simulink model "IEEE_14bus"  (R2021a)
settings: Solver=VariableStepAuto  StartTime=0.0  StopTime=16  RelTol=1e-3
undefined symbols (not defined in the file): c, cost, Discrete, linsys1, M, Mdot, Req, THeater, Time, TinIC
libraries: spsThreePhaseVIMeasurementLib x52, spsThreePhasePISectionLineLib x20, spsPMUPLLBasedPositiveSequenceLib x14, spsThreePhaseSeriesRLCLoadLib x12, spsThreePhaseTransformerTwoWindingsLib x6, simulink x6, spsThreePhaseBreakerLib x4, rllib x3, simulink_extras x3, eeStairGenerator x3, spsThreePhaseSourceLib x3, spsSynchronousMachinepuStandardLib x3
(part 2 of 3)

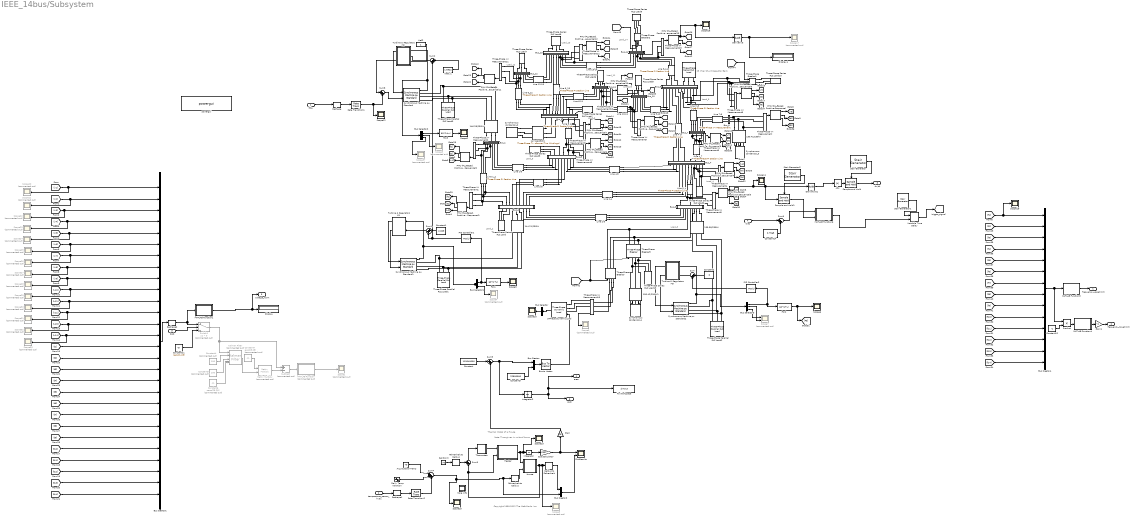
== system IEEE_14bus/Subsystem ==
  note: 25 MVar Shunt
      | Capacitor Bank
  note: Load_9
  note: Copyright 1990-2012 The MathWorks, Inc.
  note: Load_10
  note: Load_14
  note: Load_13
  note: Load_5
  note: Load_4
  note: Thermal Model of a House
  note: Load_2
  note: Load_3
  note: Load_12
  note: Load_11
  note: Note: Time given in units of hours
  note: Load_6
  fdia : Inport
  temperature_sensor_hvac : Inport  Port=2
  DoS : Inport  Port=3
  bias : Inport  Port=4
  " " : spsThreePhaseSeriesRLCLoadLib/Three-Phase Series RLC Load  LConnTagsString=A|B|C  Configuration=Y (grounded)  NominalVoltage=230e3  Vabc=[1e3 1e3 1e3]  Vabcp=[1e3 1e3 1e3]  NominalFrequency=60  UnbalancedPower=off  ActivePower=0  InductivePower=0  CapacitivePower=25e6  Pabc=[10e3 9e3 11e3]  QLabc=[100 90 110]  QCabc=[100 90 110]  Pabcp=[10e3 9e3 11e3]  QLabcp=[100 90 110]  QCabcp=[100 90 110]  Measurements=None  LoadType=constant Z
  139.38/230kV : spsThreePhaseTransformerTwoWindingsLib/Three-Phase Transformer (Two Windings)  Winding1Connection=Yg  Winding2Connection=Yg  CoreType=Three single-phase transformers  SetSaturation=off  Hysteresis=off  DataFile='hysteresis'  SetInitialFlux=off  Measurements=None  UNITS=pu  NominalPower=[ 120e6 , 60 ]  Winding1=[139.38e3 , 0.002 , 0.08 ]  Winding2=[ 230e3 , 0.002 , 0.08 ]  Rm=500  Lm=500  L0=0.5  Saturation=[ 0,0 ; 0.0024,1.2 ; 1.0,1.52 ]  InitialFluxes=[ 0.8 , -0.8 , 0.7 ]  BreakLoop=off  DiscreteSolver=Trapezoidal iterative  DataType=off  TransfoNumber=1
  144.21/230kV : spsThreePhaseTransformerTwoWindingsLib/Three-Phase Transformer (Two Windings)  Winding1Connection=Yg  Winding2Connection=Yg  CoreType=Three single-phase transformers  SetSaturation=off  Hysteresis=off  DataFile='hysteresis'  SetInitialFlux=off  Measurements=None  UNITS=pu  NominalPower=[ 120e6 , 60 ]  Winding1=[144.21e3 , 0.002 , 0.08 ]  Winding2=[ 230e3 , 0.002 , 0.08 ]  Rm=500  Lm=500  L0=0.5  Saturation=[ 0,0 ; 0.0024,1.2 ; 1.0,1.52 ]  InitialFluxes=[ 0.8 , -0.8 , 0.7 ]  BreakLoop=off  DiscreteSolver=Trapezoidal iterative  DataType=off  TransfoNumber=1
  146.28/230kV : spsThreePhaseTransformerTwoWindingsLib/Three-Phase Transformer (Two Windings)  Winding1Connection=Yg  Winding2Connection=Yg  CoreType=Three single-phase transformers  SetSaturation=off  Hysteresis=off  DataFile='hysteresis'  SetInitialFlux=off  Measurements=None  UNITS=pu  NominalPower=[ 120e6 , 60 ]  Winding1=[146.28e3 , 0.002 , 0.08 ]  Winding2=[ 230e3 , 0.002 , 0.08 ]  Rm=500  Lm=500  L0=0.5  Saturation=[ 0,0 ; 0.0024,1.2 ; 1.0,1.52 ]  InitialFluxes=[ 0.8 , -0.8 , 0.7 ]  BreakLoop=off  DiscreteSolver=Trapezoidal iterative  DataType=off  TransfoNumber=1
  147.66/230kV : spsThreePhaseTransformerTwoWindingsLib/Three-Phase Transformer (Two Windings)  Winding1Connection=Yg  Winding2Connection=Yg  CoreType=Three single-phase transformers  SetSaturation=off  Hysteresis=off  DataFile='hysteresis'  SetInitialFlux=off  Measurements=None  UNITS=pu  NominalPower=[ 120e6 , 60 ]  Winding1=[147.66e3 , 0.002 , 0.08 ]  Winding2=[ 230e3 , 0.002 , 0.08 ]  Rm=500  Lm=500  L0=0.5  Saturation=[ 0,0 ; 0.0024,1.2 ; 1.0,1.52 ]  InitialFluxes=[ 0.8 , -0.8 , 0.7 ]  BreakLoop=off  DiscreteSolver=Trapezoidal iterative  DataType=off  TransfoNumber=1
  150.42/230kV : spsThreePhaseTransformerTwoWindingsLib/Three-Phase Transformer (Two Windings)  Winding1Connection=Yg  Winding2Connection=Yg  CoreType=Three single-phase transformers  SetSaturation=off  Hysteresis=off  DataFile='hysteresis'  SetInitialFlux=off  Measurements=None  UNITS=pu  NominalPower=[ 120e6 , 60 ]  Winding1=[150.42e3 , 0.002 , 0.08 ]  Winding2=[ 230e3 , 0.002 , 0.08 ]  Rm=500  Lm=500  L0=0.5  Saturation=[ 0,0 ; 0.0024,1.2 ; 1.0,1.52 ]  InitialFluxes=[ 0.8 , -0.8 , 0.7 ]  BreakLoop=off  DiscreteSolver=Trapezoidal iterative  DataType=off  TransfoNumber=1
  150.42/230kV1 : spsThreePhaseTransformerTwoWindingsLib/Three-Phase Transformer (Two Windings)  Winding1Connection=Yg  Winding2Connection=Yg  CoreType=Three single-phase transformers  SetSaturation=off  Hysteresis=off  DataFile='hysteresis'  SetInitialFlux=off  Measurements=None  UNITS=pu  NominalPower=[ 120e6 , 60 ]  Winding1=[150.42e3 , 0.002 , 0.08 ]  Winding2=[ 230e3 , 0.002 , 0.08 ]  Rm=500  Lm=500  L0=0.5  Saturation=[ 0,0 ; 0.0024,1.2 ; 1.0,1.52 ]  InitialFluxes=[ 0.8 , -0.8 , 0.7 ]  BreakLoop=off  DiscreteSolver=Trapezoidal iterative  DataType=off  TransfoNumber=1
  3-Phase Dynamic Load : spsThreePhaseDynamicLoadLib/Three-Phase Dynamic Load  NominalVoltage=[ (217684)*1 60 ]  ActiveReactivePowers=[113.04e6 22.8e6]  PositiveSequence=[0.98441 -1.41063]  ExternalControl=on  NpNq="[1  1]"  TimeConstants="[0  0  0  0]"  MinimumVoltage=0.7  Tfilter=1e-4  LoadFlowParameters=[4 50000000 0 0 25000000]
      settings: SourceProductBaseCode=PS
  Abs : Abs
  Avg Outdoor Temp : Constant  Value=70
  Bus Creator : BusCreator  Inputs=2
  Bus Creator1 : BusCreator  Inputs=28
  Bus Creator2 : BusCreator  Inputs=2
  Bus Creator4 : BusCreator  Inputs=14
  Bus Selector : BusSelector  OutputSignals=Positive-sequence voltage V (pu)
  Bus Selector1 : BusSelector  OutputSignals="Mechanical.Rotor speed deviation  dw (pu),Mechanical.Electrical power  Pe (pu)"
  Bus Selector2 : BusSelector  OutputSignals="Mechanical.Rotor speed deviation  dw (pu),Mechanical.Electrical power  Pe (pu),dq0 components.Stator current  id (pu)"
  Bus Selector3 : BusSelector  OutputSignals="Mechanical.Rotor speed deviation  dw (pu),Mechanical.Electrical power  Pe (pu),Output active power   Peo (pu)"
  Bus to Vector : BusToVector
  Bus_1 : Subsystem
  Bus_10 : Subsystem
  Bus_11 : Subsystem
  Bus_12 : Subsystem
  Bus_13 : Subsystem
  Bus_14 : Subsystem
  Bus_2 : Subsystem
  Bus_3 : Subsystem
  Bus_4 : Subsystem
  Bus_5 : Subsystem
  Bus_6 : Subsystem
  Bus_7 : Subsystem
  Bus_8 : spsThreePhaseVIMeasurementLib/Three-Phase V-I Measurement  VoltageMeasurement=phase-to-phase  SetLabelV=on  LabelV=VB_8  Vpu=off  VpuLL=off  CurrentMeasurement=yes  SetLabelI=on  LabelI=IB_8  Ipu=off  Pbase=100e6  Vbase=500e3  OutputType=Complex  PhasorSimulation=off  PSBequivalent=0
  Bus_9 : Subsystem
  Celsius to Fahrenheit : simulink_extras/Transformations/Celsius to Fahrenheit
      settings: SourceProductBaseCode=SL
  Constant : Constant  Value=113040000
  Constant1 : Constant  Value=2.009
  Constant11 : Constant  Value=zeros(1,28)
  Constant12 : Constant  Value=-1
  Constant14 : Constant  Value=0.75e5
  Constant2 : Constant  Value=0
  Constant3 : Constant  Value=22800000
  Constant4 : Constant  Commented=on  Value=100
  Constant5 : Constant  Commented=on  Value=100
  Constant6 : Constant  Commented=on  Value=zeros(28,28)
  Constant7 : Constant  Commented=on  Value=eye(28,28)
  Cost Calculator : Gain  Gain=cost  SaturateOnIntegerOverflow=on  OutDataTypeStr=Inherit: Same as input  ParamDataTypeStr=Inherit: Same as input
  Daily Temp Variation : Sin  Amplitude=-7  Frequency=2*pi/120  SampleTime=0
  Derivative : Derivative
  Derivative1 : Derivative
  Display : Display
  Display4 : Display
  Fahrenheit to Celsius : simulink_extras/Transformations/Fahrenheit to Celsius
      settings: SourceProductBaseCode=SL
  "Fahrenheit to Celsius " : simulink_extras/Transformations/Fahrenheit to Celsius
      settings: SourceProductBaseCode=SL
  Fcn1 : Fcn  Expr=60*(1+u)
  Fcn2 : Fcn  Expr=60*(1+u)
  Fcn3 : Fcn  Expr=60*(1+u)
  Gain : Gain  Gain=9e7
  Gain1 : Gain  Gain=-1
  Heater : Subsystem
  House : Subsystem
      mask Display: image(fullfile(matlabroot,'toolbox','simulink','simdemos','simgeneral','images','HouseHeatHousePix.svg'))
  Integrator : Integrator  InitialCondition=TinIC
  Integrator2 : Integrator
  Kalman Filter : ctrlSharedLib/Kalman Filter  Commented=on  TimeDomain=Discrete-Time  UseCurrentEstimator=on  ModelSource=Individual A, B, C, D matrices  ModelSourceVariable=ss(0.95,1,1,0,1)  A=eye(28,28)  B=linsys1.B  C=eye(28,28)  D=linsys1.D  NumberOfStates=1  NumberOfInputs=1  NumberOfOutputs=1  InitialEstimateSource=Dialog  X0=0  P0=10  UseK=off  UseGH=off  NumberOfProcessNoiseInputs=1  G=1  TimeInvariantG=on  H=0  TimeInvariantH=on  Q=0.05  TimeInvariantQ=off  R=1  TimeInvariantR=off  N=0  TimeInvariantN=off  AddInputPort=off  AddEnablePort=off  OutputEstimatedY=off  OutputP=off  Ts=-1
  Line 1-5 : spsThreePhasePISectionLineLib/Three-Phase PI Section Line  LConnTagsString=a|b|c  RConnTagsString=A|B|C  Length=78.64  Frequency=60  Resistances=[ 0.3029 0.9086]  Inductances=[ 0.0033 0.0099]  Capacitances=[3.35e-9 1.01e-8]
  Line 10-11 : spsThreePhasePISectionLineLib/Three-Phase PI Section Line  LConnTagsString=a|b|c  RConnTagsString=A|B|C  Length=4.93  Frequency=60  Resistances=[ 0.3667 1.1002]  Inductances=[ 0.0023 0.0068]  Capacitances=[1.22e-11 3.66e-11]
  Line 12-13 : spsThreePhasePISectionLineLib/Three-Phase PI Section Line  LConnTagsString=a|b|c  RConnTagsString=A|B|C  Length=5.03  Frequency=60  Resistances=[ 0.9679 2.9038]  Inductances=[ 0.0023 0.0070]  Capacitances=[1.20e-11 3.59e-11]
  Line 13-14 : spsThreePhasePISectionLineLib/Three-Phase PI Section Line  LConnTagsString=a|b|c  RConnTagsString=A|B|C  Length=6.64  Frequency=60  Resistances=[ 0.5676 1.7027]  Inductances=[ 0.0031 0.0092]  Capacitances=[9.06e-12 2.72e-11]
  Line 1_2 : spsThreePhasePISectionLineLib/Three-Phase PI Section Line  LConnTagsString=a|b|c  RConnTagsString=A|B|C  Length=44.47  Frequency=60  Resistances=[ 0.1921 0.5763]  Inductances=[ 0.0016 0.0047]  Capacitances=[7.14e-9 2.14e-8]
  Line 2-3 : spsThreePhasePISectionLineLib/Three-Phase PI Section Line  LConnTagsString=a|b|c  RConnTagsString=A|B|C  Length=68.47  Frequency=60  Resistances=[ 0.3026 0.9077]  Inductances=[ 0.0034 0.0101]  Capacitances=[3.29e-9 9.86e-8]
  Line 2-4 : spsThreePhasePISectionLineLib/Three-Phase PI Section Line  LConnTagsString=a|b|c  RConnTagsString=A|B|C  Length=74.11  Frequency=60  Resistances=[ 0.3457 1.0370]  Inductances=[ 0.0028 0.0083]  Capacitances=[3.99e-9 1.20e-8]
  Line 2-5 : spsThreePhasePISectionLineLib/Three-Phase PI Section Line  LConnTagsString=a|b|c  RConnTagsString=A|B|C  Length=61.18  Frequency=60  Resistances=[ 0.4104 1.2311]  Inductances=[ 0.0033 0.0100]  Capacitances=[3.34e-9 1.0e-8]
  Line 3_4 : spsThreePhasePISectionLineLib/Three-Phase PI Section Line  LConnTagsString=a|b|c  RConnTagsString=A|B|C  Length=61.21  Frequency=60  Resistances=[ 0.4826 1.4479]  Inductances=[ 0.0033 0.0098]  Capacitances=[3.4e-9 1.02e-8]
  Line 4-5 : spsThreePhasePISectionLineLib/Three-Phase PI Section Line  LConnTagsString=a|b|c  RConnTagsString=A|B|C  Length=18.47  Frequency=60  Resistances=[ 0.3186 0.9558]  Inductances=[ 0.0027 0.0080]  Capacitances=[4.17e-9 1.25e-8]
  Line 4_7 : spsThreePhasePISectionLineLib/Three-Phase PI Section Line  LConnTagsString=a|b|c  RConnTagsString=A|B|C  Length=5.15  Frequency=60  Resistances=[ 0.0001 0.0003]  Inductances=[ 0.0475 0.1425]  Capacitances=[2.34e-10 7.02e-10]
  Line 4_9 : spsThreePhasePISectionLineLib/Three-Phase PI Section Line  LConnTagsString=a|b|c  RConnTagsString=A|B|C  Length=8.39  Frequency=60  Resistances=[ 0.0001 0.0003]  Inductances=[ 0.0775 0.2325]  Capacitances=[1.43e-10 4.3e-10]
  Line 5_6 : spsThreePhasePISectionLineLib/Three-Phase PI Section Line  LConnTagsString=a|b|c  RConnTagsString=A|B|C  Length=5.65  Frequency=60  Resistances=[ 0.0001 0.0003]  Inductances=[ 0.0522 0.1565]  Capacitances=[2.13e-10 6.39e-10]
  Line 6-11 : spsThreePhasePISectionLineLib/Three-Phase PI Section Line  LConnTagsString=a|b|c  RConnTagsString=A|B|C  Length=5.02  Frequency=60  Resistances=[ 0.4172 1.2515]  Inductances=[ 0.0023 0.0070]  Capacitances=[1.20e-11 3.60e-11]
  Line 6_12 : spsThreePhasePISectionLineLib/Three-Phase PI Section Line  LConnTagsString=a|b|c  RConnTagsString=A|B|C  Length=5.69  Frequency=60  Resistances=[ 0.4760 1.4281]  Inductances=[ 0.0026 0.0079]  Capacitances=[1.06e-11 3.17e-11]
  Line 6_13 : spsThreePhasePISectionLineLib/Three-Phase PI Section Line  LConnTagsString=a|b|c  RConnTagsString=A|B|C  Length=4.06  Frequency=60  Resistances=[ 0.3590 1.0770]  Inductances=[ 0.0019 0.0056]  Capacitances=[1.48e-11 4.44e-11]
  Line 7-8 : spsThreePhasePISectionLineLib/Three-Phase PI Section Line  LConnTagsString=a|b|c  RConnTagsString=A|B|C  Length=4.72  Frequency=60  Resistances=[ 0.0005 0.0014]  Inductances=[ 0.0022 0.0065]  Capacitances=[ 1.27e-11 3.82e-11]
  Line 7_9 : spsThreePhasePISectionLineLib/Three-Phase PI Section Line  LConnTagsString=a|b|c  RConnTagsString=A|B|C  Length=3.73  Frequency=60  Resistances=[ 0.0006 0.0018]  Inductances=[ 0.0017 0.0052]  Capacitances=[ 1.61e-11 4.84e-11]
  Line 9-10 : spsThreePhasePISectionLineLib/Three-Phase PI Section Line  LConnTagsString=a|b|c  RConnTagsString=A|B|C  Length=3.27  Frequency=60  Resistances=[ 0.2144 0.6431]  Inductances=[ 0.0015 0.0045]  Capacitances=[1.84e-11 5.52e-11]
  Line 9_14 : spsThreePhasePISectionLineLib/Three-Phase PI Section Line  LConnTagsString=a|b|c  RConnTagsString=A|B|C  Length=5.85  Frequency=60  Resistances=[ 0.4788 1.4365]  Inductances=[ 0.0027 0.0081]  Capacitances=[1.03e-11 3.08e-11]
  MATLAB Function : MATLAB Function  Commented=on  TreatAsAtomicUnit=on
  MATLAB Function1 : MATLAB Function  TreatAsAtomicUnit=on
  MATLAB Function3 : MATLAB Function  TreatAsAtomicUnit=on
  MATLAB Function4 : MATLAB Function  TreatAsAtomicUnit=on
  MATLAB Function6 : MATLAB Function  TreatAsAtomicUnit=on
  Matrix Multiply : Product  Commented=on  Multiplication=Matrix(*)
  More Info : Subsystem
      settings: OpenFcn=showExample('simulink_general/sldemo_househeatExample')
      mask Display: disp('?')
  PID Controller1 : slpidlib/PID Controller  Controller=PID  Form=Parallel  TimeDomain=Discrete-time  UseExternalTs=off  SampleTime=-1  IntegratorMethod=Forward Euler  FilterMethod=Forward Euler  ControllerParametersSource=internal  P=-2.009  I=10  D=0  UseFilter=on  N=100  TunerSelectOption=Frequency Response Based  InitialConditionSource=internal  InitialConditionForIntegrator=0  InitialConditionForFilter=0  DifferentiatorICPrevScaledInput=0  ExternalReset=none  TrackingMode=off  Kt=1  LimitOutput=off  SatLimitsSource=internal  UpperSaturationLimit=inf  LowerSaturationLimit=-inf  LinearizeAsGain=on  AntiWindupMode=none  Kb=1  POutMin=[]  POutMax=[]  IOutMin=[]  IOutMax=[]  DOutMin=[]  DOutMax=[]  NOutMin=[]  NOutMax=[]  SumOutMin=[]  SumOutMax=[]  SaturationOutMin=[]  SaturationOutMax=[]  PParamMin=[]  PParamMax=[]  IParamMin=[]  IParamMax=[]  DParamMin=[]  DParamMax=[]  NParamMin=[]  NParamMax=[]  KbParamMin=[]  KbParamMax=[]  KtParamMin=[]  KtParamMax=[]  KbOutMin=[]  KbOutMax=[]  KtOutMin=[]  KtOutMax=[]  IntegratorOutMin=[]  IntegratorOutMax=[]  FilterOutMin=[]  FilterOutMax=[]  SumI1OutMin=[]  SumI1OutMax=[]  SumI2OutMin=[]  SumI2OutMax=[]  SumI3OutMin=[]  SumI3OutMax=[]  SumI4OutMin=[]  SumI4OutMax=[]  SumDOutMin=[]  SumDOutMax=[]  DifferentiatorOutMin=[]  DifferentiatorOutMax=[]  FilterDiffOutCoefMin=[]  FilterDiffOutCoefMax=[]  ReciprocalOutMin=[]  ReciprocalOutMax=[]  SumDenOutMin=[]  SumDenOutMax=[]  SumNumOutMin=[]  SumNumOutMax=[]  DivideOutMin=[]  DivideOutMax=[]  UdiffTsProdOutMin=[]  UdiffTsProdOutMax=[]  NTsProdOutMin=[]  NTsProdOutMax=[]  UintegralTsProdOutMin=[]  UintegralTsProdOutMax=[]  UngainTsProdOutMin=[]  UngainTsProdOutMax=[]  IntegratorContinuousStateAttributes=''  IntegratorStateMustResolveToSignalObject=off  IntegratorRTWStateStorageClass=Auto  FilterContinuousStateAttributes=''  FilterStateMustResolveToSignalObject=off  FilterRTWStateStorageClass=Auto  ParallelPVariant=InternalParameters  IdealPVariant=Disabled  IVariant=InternalParameters  DVariant=InternalParameters  IntegratorVariant=Discrete  SatVariant=Disabled  AWVariant=Passthrough  PCopyVariant=Disabled  TRVariant=Disabled  FdbkBlocksVariant=Forward  IdealPFdbkVariant=Disabled  SatFdbkVariant=Disabled  DerivativeFilterVariant=ForwardEulerFilter  NVariant=InternalParameters  NCopyVariant=Disabled  FilterICVariant=InternalICsFilter  IntegratorICVariant=InternalICs  ExternalResetVariant=Disabled  TRSumVariant=Passthrough  SumFdbkVariant=Disabled  SumVariant=Sum_PID  TsampFilterVariant=InternalTs  TsampNgainVariant=Passthrough  TsampIntegralVariant=Passthrough  ExternalSaturationOutDataTypeStr=Inherit: Same as second input
  PID Controller2 : slpidlib/PID Controller  Controller=PID  Form=Parallel  TimeDomain=Discrete-time  UseExternalTs=off  SampleTime=-1  IntegratorMethod=Forward Euler  FilterMethod=Forward Euler  ControllerParametersSource=internal  P=-2  I=10  D=0  UseFilter=on  N=100  TunerSelectOption=Transfer Function Based (PID Tuner App)  InitialConditionSource=internal  InitialConditionForIntegrator=0  InitialConditionForFilter=0  DifferentiatorICPrevScaledInput=0  ExternalReset=none  TrackingMode=off  Kt=1  LimitOutput=off  SatLimitsSource=internal  UpperSaturationLimit=inf  LowerSaturationLimit=-inf  LinearizeAsGain=on  AntiWindupMode=none  Kb=1  POutMin=[]  POutMax=[]  IOutMin=[]  IOutMax=[]  DOutMin=[]  DOutMax=[]  NOutMin=[]  NOutMax=[]  SumOutMin=[]  SumOutMax=[]  SaturationOutMin=[]  SaturationOutMax=[]  PParamMin=[]  PParamMax=[]  IParamMin=[]  IParamMax=[]  DParamMin=[]  DParamMax=[]  NParamMin=[]  NParamMax=[]  KbParamMin=[]  KbParamMax=[]  KtParamMin=[]  KtParamMax=[]  KbOutMin=[]  KbOutMax=[]  KtOutMin=[]  KtOutMax=[]  IntegratorOutMin=[]  IntegratorOutMax=[]  FilterOutMin=[]  FilterOutMax=[]  SumI1OutMin=[]  SumI1OutMax=[]  SumI2OutMin=[]  SumI2OutMax=[]  SumI3OutMin=[]  SumI3OutMax=[]  SumI4OutMin=[]  SumI4OutMax=[]  SumDOutMin=[]  SumDOutMax=[]  DifferentiatorOutMin=[]  DifferentiatorOutMax=[]  FilterDiffOutCoefMin=[]  FilterDiffOutCoefMax=[]  ReciprocalOutMin=[]  ReciprocalOutMax=[]  SumDenOutMin=[]  SumDenOutMax=[]  SumNumOutMin=[]  SumNumOutMax=[]  DivideOutMin=[]  DivideOutMax=[]  UdiffTsProdOutMin=[]  UdiffTsProdOutMax=[]  NTsProdOutMin=[]  NTsProdOutMax=[]  UintegralTsProdOutMin=[]  UintegralTsProdOutMax=[]  UngainTsProdOutMin=[]  UngainTsProdOutMax=[]  IntegratorContinuousStateAttributes=''  IntegratorStateMustResolveToSignalObject=off  IntegratorRTWStateStorageClass=Auto  FilterContinuousStateAttributes=''  FilterStateMustResolveToSignalObject=off  FilterRTWStateStorageClass=Auto  ParallelPVariant=InternalParameters  IdealPVariant=Disabled  IVariant=InternalParameters  DVariant=InternalParameters  IntegratorVariant=Discrete  SatVariant=Disabled  AWVariant=Passthrough  PCopyVariant=Disabled  TRVariant=Disabled  FdbkBlocksVariant=Forward  IdealPFdbkVariant=Disabled  SatFdbkVariant=Disabled  DerivativeFilterVariant=ForwardEulerFilter  NVariant=InternalParameters  NCopyVariant=Disabled  FilterICVariant=InternalICsFilter  IntegratorICVariant=InternalICs  ExternalResetVariant=Disabled  TRSumVariant=Passthrough  SumFdbkVariant=Disabled  SumVariant=Sum_PID  TsampFilterVariant=InternalTs  TsampNgainVariant=Passthrough  TsampIntegralVariant=Passthrough  ExternalSaturationOutDataTypeStr=Inherit: Same as second input
  PMU (PLL-Based, Positive-Sequence){,1..13} (14 alike) : spsPMUPLLBasedPositiveSequenceLib/PMU (PLL-Based, Positive-Sequence)  nominalFrequency=60  samplingRate=64  reportingFactor=1
      settings: SourceProductBaseCode=PS
  PlotResults : Scope  NumInputPorts=2
  Product : Product
  Rate Transition1 : RateTransition
  Rate Transition2 : RateTransition
  Reshape : Reshape
  Reshape1 : Reshape
  Reshape2 : Reshape
  Sample and Hold : dspsigops/Sample and Hold  trig=Rising edge  initCond=0  latchinput=off
  Sample and Hold1 : dspsigops/Sample and Hold  trig=Rising edge  initCond=0  latchinput=off
  Scope{1,4..5,8..9,17,20..33,37} (21 alike) : Scope  Commented=on
  Scope{2..3,6,10..13,15..16,19} (10 alike) : Scope
  Scope7 : Scope  Commented=on  NumInputPorts=2
  Set Point : Constant  Value=70
  Stair Generator : eeStairGenerator/Stair Generator  LabelModeActiveChoice=Discrete  TimeInput=[0 5 10 15 20 25 30 35 40 45 50]  AmplitudeInput=[0 1 0 1 0 1 0 1 0 1 0 ]  SampleTime=5e-5  RepeatPattern=off  OutDataTypeStr=double
      settings: SourceProductBaseCode=PS
  Stair Generator1 : eeStairGenerator/Stair Generator  LabelModeActiveChoice=Discrete  TimeInput=[0 5 60]  AmplitudeInput=[0 1 1 ]  SampleTime=5e-5  RepeatPattern=off  OutDataTypeStr=double
      settings: SourceProductBaseCode=PS
  Stair Generator2 : eeStairGenerator/Stair Generator  LabelModeActiveChoice=Discrete  TimeInput=[0 5 10 15 20 25 30 35 40 45 50]  AmplitudeInput="[0 1 0 1 0 1 0 1 0 1 0  ]"  SampleTime=5e-5  RepeatPattern=off  OutDataTypeStr=double
      settings: SourceProductBaseCode=PS
  Subtract : Sum  Commented=on  Inputs=+-
  Sum{,1..2,5,8..9} (6 alike) : Sum  Inputs=|++
  Sum3 : Sum  Inputs=+-|  InputSameDT=on  SaturateOnIntegerOverflow=on  OutDataTypeStr=Inherit: Same as first input
  Sum4 : Sum  Inputs=|+++
  Switch1 : Switch  Commented=on  Criteria=u2 > Threshold
  Synchronous condensor_1 : spsThreePhaseSourceLib/Three-Phase Source  InternalConnection=Yg  VoltagePhases=off  Voltage=(150420)*0.995122  PhaseAngle=-36.1424  Voltage_phases=[25e3 25e3 25e3]/sqrt(3)  PhaseAngles_phases=[0 -120 +120]  Frequency=60  NonIdealSource=on  SpecifyImpedance=off  Resistance=0.8929  Inductance=16.58e-3  ShortCircuitLevel=100e6  BaseVoltage=150.42e3  XRratio=7  BusType=PQ  Pref=0  Qref=30.144e6  Prefabc=[10e3, 10e3, 10e3]  Qrefabc=[0, 0, 0]  Qmin=-inf  Qmax=inf
  Synchronous condensor_2 : spsThreePhaseSourceLib/Three-Phase Source  InternalConnection=Yg  VoltagePhases=off  Voltage=(147660)*0.984306  PhaseAngle=-36.2022  Voltage_phases=[25e3 25e3 25e3]/sqrt(3)  PhaseAngles_phases=[0 -120 +120]  Frequency=60  NonIdealSource=on  SpecifyImpedance=off  Resistance=0.8929  Inductance=16.58e-3  ShortCircuitLevel=100e6  BaseVoltage=147.66e3  XRratio=7  BusType=PQ  Pref=0  Qref=25.276e6  Prefabc=[10e3, 10e3, 10e3]  Qrefabc=[0, 0, 0]  Qmin=-inf  Qmax=inf
  Synchronous condensor_3 : spsThreePhaseSourceLib/Three-Phase Source  InternalConnection=Yg  VoltagePhases=off  Voltage=(150420)*0.995122  PhaseAngle=-36.1424  Voltage_phases=[25e3 25e3 25e3]/sqrt(3)  PhaseAngles_phases=[0 -120 +120]  Frequency=60  NonIdealSource=on  SpecifyImpedance=off  Resistance=0.8929  Inductance=16.58e-3  ShortCircuitLevel=100e6  BaseVoltage=150.42e3  XRratio=7  BusType=PQ  Pref=0  Qref=30.144e6  Prefabc=[10e3, 10e3, 10e3]  Qrefabc=[0, 0, 0]  Qmin=-inf  Qmax=inf
  Synchronous Machine pu Standard : spsSynchronousMachinepuStandardLib/Synchronous Machine pu Standard  PresetModel=No  MechanicalLoad=Mechanical power Pm  ShowDetailedParameters=on  RotorType=Salient-pole  Units=per unit standard parameters  MeasurementBus=off  NominalParameters="[90E6  146280   60 ]"  Reactances1=[ 1.81, 0.3, 0.23, 1.76, 0.65, 0.25, 0.15 ]  Reactances2=[ 1.305, 0.296, 0.252, 0.474, 0.243, 0.18 ]  dAxisTimeConstants=Short-circuit  qAxisTimeConstants=Open-circuit  TimeConstants1="[ 4.4849  0.0681  0.1  ]"  TimeConstants2=[ 8.0, 0.03, 1.0, 0.07 ]  TimeConstants3="[  4.49  0.0681  0.0513  ]"  TimeConstants4=[ 8.0, 0.03, 0.3371, 0.0295 ]  TimeConstants5=[ 1.01, 0.053, 0.1 ]  TimeConstants6=[ 1.3201, 0.023, 1.0, 0.07 ]  TimeConstants7=[0.012 0.003 0.003]  TimeConstants8=[ 1.3201, 0.0231, 0.3371, 0.0295 ]  StatorResistance=2.8544e-3  Mechanical="[ 3.7 0  32]"  PolePairs=20  InitialConditions=[0 -55.1684 1.72023 1.72023 1.72023 -10.3587 -130.359 109.641 2.41694]  SetSaturation=off  Saturation=[0.6404,0.7127,0.8441,0.9214,0.9956,1.082,1.19,1.316,1.457;0.7,0.7698,0.8872,0.9466,0.9969,1.046,1.1,1.151,1.201]  LoadFlowParameters=[1 0 0 0 0]  TsPowergui=0  TsBlock=-1  IterativeModel=Trapezoidal non iterative  IterativeDiscreteModel=Trapezoidal non iterative  BusType=swing  Pref=0  Qref=0  Qmin=-inf  Qmax=inf  PLF=0  QLF=0
      settings: SourceProductBaseCode=PS
  Synchronous Machine pu Standard1 : spsSynchronousMachinepuStandardLib/Synchronous Machine pu Standard  PresetModel=No  MechanicalLoad=Mechanical power Pm  ShowDetailedParameters=on  RotorType=Salient-pole  Units=per unit standard parameters  MeasurementBus=off  NominalParameters="[90E6  144210   60 ]"  Reactances1=[ 1.81, 0.3, 0.23, 1.76, 0.65, 0.25, 0.15 ]  Reactances2=[ 1.305, 0.296, 0.252, 0.474, 0.243, 0.18 ]  dAxisTimeConstants=Short-circuit  qAxisTimeConstants=Open-circuit  TimeConstants1="[ 4.4849  0.0681  0.1  ]"  TimeConstants2=[ 8.0, 0.03, 1.0, 0.07 ]  TimeConstants3="[  4.49  0.0681  0.0513  ]"  TimeConstants4=[ 8.0, 0.03, 0.3371, 0.0295 ]  TimeConstants5=[ 1.01, 0.053, 0.1 ]  TimeConstants6=[ 1.3201, 0.023, 1.0, 0.07 ]  TimeConstants7=[0.012 0.003 0.003]  TimeConstants8=[ 1.3201, 0.0231, 0.3371, 0.0295 ]  StatorResistance=2.8544e-3  Mechanical="[ 3.7 0  32]"  PolePairs=20  InitialConditions=[0 -52.2742 2.06355 2.06355 2.06355 -13.2061 -133.206 106.794 2.88545]  SetSaturation=off  Saturation=[0.6404,0.7127,0.8441,0.9214,0.9956,1.082,1.19,1.316,1.457;0.7,0.7698,0.8872,0.9466,0.9969,1.046,1.1,1.151,1.201]  LoadFlowParameters=[1,0,0,0,0]  TsPowergui=0  TsBlock=-1  IterativeModel=Trapezoidal non iterative  IterativeDiscreteModel=Trapezoidal non iterative  BusType=swing  Pref=0  Qref=0  Qmin=-inf  Qmax=inf  PLF=0  QLF=0
      settings: SourceProductBaseCode=PS
  Synchronous Machine pu Standard2 : spsSynchronousMachinepuStandardLib/Synchronous Machine pu Standard  PresetModel=No  MechanicalLoad=Mechanical power Pm  ShowDetailedParameters=on  RotorType=Salient-pole  Units=per unit standard parameters  MeasurementBus=off  NominalParameters="[90E6  139380  60 ]"  Reactances1=[ 1.81, 0.3, 0.23, 1.76, 0.65, 0.25, 0.15 ]  Reactances2=[ 1.305, 0.296, 0.252, 0.474, 0.243, 0.18 ]  dAxisTimeConstants=Short-circuit  qAxisTimeConstants=Open-circuit  TimeConstants1="[ 4.4849  0.0681  0.1  ]"  TimeConstants2=[ 8.0, 0.03, 1.0, 0.07 ]  TimeConstants3="[  4.49  0.0681  0.0513  ]"  TimeConstants4=[ 8.0, 0.03, 0.3371, 0.0295 ]  TimeConstants5=[ 1.01, 0.053, 0.1 ]  TimeConstants6=[ 1.3201, 0.023, 1.0, 0.07 ]  TimeConstants7=[0.012 0.003 0.003]  TimeConstants8=[ 1.3201, 0.0231, 0.3371, 0.0295 ]  StatorResistance=2.8544e-3  Mechanical="[ 3.7 0  32]"  PolePairs=20  InitialConditions=[0 -114.329 0.550177 0.550177 0.550177 -114.259 -234.259 5.74123 1.7297]  SetSaturation=off  Saturation=[0.6404,0.7127,0.8441,0.9214,0.9956,1.082,1.19,1.316,1.457;0.7,0.7698,0.8872,0.9466,0.9969,1.046,1.1,1.151,1.201]  LoadFlowParameters=[1,0,0,0,0]  TsPowergui=0  TsBlock=-1  IterativeModel=Trapezoidal non iterative  IterativeDiscreteModel=Trapezoidal non iterative  BusType=PV  Pref=1e10  Qref=0  Qmin=50096006  Qmax=50096006  PLF=0  QLF=0
      settings: SourceProductBaseCode=PS
  Thermostat : Subsystem
      mask Display: image(fullfile(matlabroot,'toolbox','simulink','simdemos','simgeneral','images','HouseHeatThermostatPix.svg'))
  Three-Phase Parallel RLC Load1 : spsThreePhaseParallelRLCLoadLib/Three-Phase Parallel RLC Load  LConnTagsString=A|B|C  Configuration=Y (grounded)  NominalVoltage=10000  Vabc=[1e3 1e3 1e3]  Vabcp=[1e3 1e3 1e3]  NominalFrequency=60  UnbalancedPower=off  ActivePower=10e3  InductivePower=2000  CapacitivePower=0  Pabc=[10e3 9e3 11e3]  QLabc=[100 90 110]  QCabc=[100 90 110]  Pabcp=[10e3 9e3 11e3]  QLabcp=[100 90 110]  QCabcp=[100 90 110]  Measurements=None  LoadType=constant Z
  Three-Phase Parallel RLC Load2 : spsThreePhaseParallelRLCLoadLib/Three-Phase Parallel RLC Load  LConnTagsString=A|B|C  Configuration=Y (grounded)  NominalVoltage=10000  Vabc=[1e3 1e3 1e3]  Vabcp=[1e3 1e3 1e3]  NominalFrequency=60  UnbalancedPower=off  ActivePower=10e3  InductivePower=2000  CapacitivePower=0  Pabc=[10e3 9e3 11e3]  QLabc=[100 90 110]  QCabc=[100 90 110]  Pabcp=[10e3 9e3 11e3]  QLabcp=[100 90 110]  QCabcp=[100 90 110]  Measurements=None  LoadType=constant Z
  Three-Phase Parallel RLC Load3 : spsThreePhaseParallelRLCLoadLib/Three-Phase Parallel RLC Load  LConnTagsString=A|B|C  Configuration=Y (grounded)  NominalVoltage=10000  Vabc=[1e3 1e3 1e3]  Vabcp=[1e3 1e3 1e3]  NominalFrequency=60  UnbalancedPower=off  ActivePower=10e3  InductivePower=2000  CapacitivePower=0  Pabc=[10e3 9e3 11e3]  QLabc=[100 90 110]  QCabc=[100 90 110]  Pabcp=[10e3 9e3 11e3]  QLabcp=[100 90 110]  QCabcp=[100 90 110]  Measurements=None  LoadType=constant Z
  Three-Phase Series RLC Load : spsThreePhaseSeriesRLCLoadLib/Three-Phase Series RLC Load  LConnTagsString=A|B|C  Configuration=Y (grounded)  NominalVoltage=(230000)*0.949726  Vabc=[1e3 1e3 1e3]  Vabcp=[1e3 1e3 1e3]  NominalFrequency=60  UnbalancedPower=off  ActivePower=26.04e6  InductivePower=15.24e6  CapacitivePower=0  Pabc=[10e3 9e3 11e3]  QLabc=[100 90 110]  QCabc=[100 90 110]  Pabcp=[10e3 9e3 11e3]  QLabcp=[100 90 110]  QCabcp=[100 90 110]  Measurements=None  LoadType=constant PQ
  Three-Phase Series RLC Load10 : spsThreePhaseSeriesRLCLoadLib/Three-Phase Series RLC Load  LConnTagsString=A|B|C  Configuration=Y (grounded)  NominalVoltage=(230000)*0.942986  Vabc=[1e3 1e3 1e3]  Vabcp=[1e3 1e3 1e3]  NominalFrequency=60  UnbalancedPower=off  ActivePower=35.4e6  InductivePower=19.92e6  CapacitivePower=0  Pabc=[10e3 9e3 11e3]  QLabc=[100 90 110]  QCabc=[100 90 110]  Pabcp=[10e3 9e3 11e3]  QLabcp=[100 90 110]  QCabcp=[100 90 110]  Measurements=None  LoadType=constant PQ
  Three-Phase Series RLC Load13 : spsThreePhaseSeriesRLCLoadLib/Three-Phase Series RLC Load  LConnTagsString=A|B|C  Configuration=Y (grounded)  NominalVoltage=(217684)*1  Vabc=[1e3 1e3 1e3]  Vabcp=[1e3 1e3 1e3]  NominalFrequency=60  UnbalancedPower=off  ActivePower=113040000  InductivePower=22800000  CapacitivePower=0  Pabc=[10e3 9e3 11e3]  QLabc=[100 90 110]  QCabc=[100 90 110]  Pabcp=[10e3 9e3 11e3]  QLabcp=[100 90 110]  QCabcp=[100 90 110]  Measurements=None  LoadType=constant PQ
  Three-Phase Series RLC Load2 : spsThreePhaseSeriesRLCLoadLib/Three-Phase Series RLC Load  LConnTagsString=A|B|C  Configuration=Y (grounded)  NominalVoltage=(230000)*0.927953  Vabc=[1e3 1e3 1e3]  Vabcp=[1e3 1e3 1e3]  NominalFrequency=60  UnbalancedPower=off  ActivePower=57.36e6  InductivePower=0  CapacitivePower=4.68e6  Pabc=[10e3 9e3 11e3]  QLabc=[100 90 110]  QCabc=[100 90 110]  Pabcp=[10e3 9e3 11e3]  QLabcp=[100 90 110]  QCabcp=[100 90 110]  Measurements=None  LoadType=constant PQ
  Three-Phase Series RLC Load3 : spsThreePhaseSeriesRLCLoadLib/Three-Phase Series RLC Load  LConnTagsString=A|B|C  Configuration=Y (grounded)  NominalVoltage=(230000)*0.931217  Vabc=[1e3 1e3 1e3]  Vabcp=[1e3 1e3 1e3]  NominalFrequency=60  UnbalancedPower=off  ActivePower=9.12e6  InductivePower=1.92e6  CapacitivePower=0  Pabc=[10e3 9e3 11e3]  QLabc=[100 90 110]  QCabc=[100 90 110]  Pabcp=[10e3 9e3 11e3]  QLabcp=[100 90 110]  QCabcp=[100 90 110]  Measurements=None  LoadType=constant PQ
  Three-Phase Series RLC Load4 : spsThreePhaseSeriesRLCLoadLib/Three-Phase Series RLC Load  LConnTagsString=A|B|C  Configuration=Y (grounded)  NominalVoltage=(230000)*0.942548  Vabc=[1e3 1e3 1e3]  Vabcp=[1e3 1e3 1e3]  NominalFrequency=60  UnbalancedPower=off  ActivePower=13.44e6  InductivePower=9e6  CapacitivePower=0  Pabc=[10e3 9e3 11e3]  QLabc=[100 90 110]  QCabc=[100 90 110]  Pabcp=[10e3 9e3 11e3]  QLabcp=[100 90 110]  QCabcp=[100 90 110]  Measurements=None  LoadType=constant PQ
  Three-Phase Series RLC Load5 : spsThreePhaseSeriesRLCLoadLib/Three-Phase Series RLC Load  LConnTagsString=A|B|C  Configuration=Y (grounded)  NominalVoltage=(230000)*0.942502  Vabc=[1e3 1e3 1e3]  Vabcp=[1e3 1e3 1e3]  NominalFrequency=60  UnbalancedPower=off  ActivePower=10.8e6  InductivePower=6.96e6  CapacitivePower=0  Pabc=[10e3 9e3 11e3]  QLabc=[100 90 110]  QCabc=[100 90 110]  Pabcp=[10e3 9e3 11e3]  QLabcp=[100 90 110]  QCabcp=[100 90 110]  Measurements=None  LoadType=constant PQ
  Three-Phase Series RLC Load6 : spsThreePhaseSeriesRLCLoadLib/Three-Phase Series RLC Load  LConnTagsString=A|B|C  Configuration=Y (grounded)  NominalVoltage=(230000)*0.942338  Vabc=[1e3 1e3 1e3]  Vabcp=[1e3 1e3 1e3]  NominalFrequency=60  UnbalancedPower=off  ActivePower=4.2e6  InductivePower=2.16e6  CapacitivePower=0  Pabc=[10e3 9e3 11e3]  QLabc=[100 90 110]  QCabc=[100 90 110]  Pabcp=[10e3 9e3 11e3]  QLabcp=[100 90 110]  QCabcp=[100 90 110]  Measurements=None  LoadType=constant PQ
  Three-Phase Series RLC Load7 : spsThreePhaseSeriesRLCLoadLib/Three-Phase Series RLC Load  LConnTagsString=A|B|C  Configuration=Y (grounded)  NominalVoltage=(230000)*0.941818  Vabc=[1e3 1e3 1e3]  Vabcp=[1e3 1e3 1e3]  NominalFrequency=60  UnbalancedPower=off  ActivePower=7.32e6  InductivePower=1.92e6  CapacitivePower=0  Pabc=[10e3 9e3 11e3]  QLabc=[100 90 110]  QCabc=[100 90 110]  Pabcp=[10e3 9e3 11e3]  QLabcp=[100 90 110]  QCabcp=[100 90 110]  Measurements=None  LoadType=constant PQ
  Three-Phase Series RLC Load8 : spsThreePhaseSeriesRLCLoadLib/Three-Phase Series RLC Load  LConnTagsString=A|B|C  Configuration=Y (grounded)  NominalVoltage=(230000)*0.941642  Vabc=[1e3 1e3 1e3]  Vabcp=[1e3 1e3 1e3]  NominalFrequency=60  UnbalancedPower=off  ActivePower=16.2e6  InductivePower=6.96e6  CapacitivePower=0  Pabc=[10e3 9e3 11e3]  QLabc=[100 90 110]  QCabc=[100 90 110]  Pabcp=[10e3 9e3 11e3]  QLabcp=[100 90 110]  QCabcp=[100 90 110]  Measurements=None  LoadType=constant PQ
  Three-Phase Series RLC Load9 : spsThreePhaseSeriesRLCLoadLib/Three-Phase Series RLC Load  LConnTagsString=A|B|C  Configuration=Y (grounded)  NominalVoltage=(230000)*0.941422  Vabc=[1e3 1e3 1e3]  Vabcp=[1e3 1e3 1e3]  NominalFrequency=60  UnbalancedPower=off  ActivePower=17.88e6  InductivePower=6e6  CapacitivePower=0  Pabc=[10e3 9e3 11e3]  QLabc=[100 90 110]  QCabc=[100 90 110]  Pabcp=[10e3 9e3 11e3]  QLabcp=[100 90 110]  QCabcp=[100 90 110]  Measurements=None  LoadType=constant PQ
  Three-Phase V-I Measurement{,1..13,15} (15 alike) : spsThreePhaseVIMeasurementLib/Three-Phase V-I Measurement  VoltageMeasurement=phase-to-ground  SetLabelV=off  LabelV=Vabc  Vpu=off  VpuLL=off  CurrentMeasurement=yes  SetLabelI=off  LabelI=Iabc  Ipu=off  Pbase=100e6  Vbase=500e3  OutputType=Complex  PhasorSimulation=off  PSBequivalent=0
  Three-Phase Breaker : spsThreePhaseBreakerLib/Three-Phase Breaker  InitialState=closed  SwitchA=on  SwitchB=on  SwitchC=on  SwitchTimes=[100]  External=on  BreakerResistance=0.01  SnubberResistance=1e6  SnubberCapacitance=inf  Measurements=None
  Three-Phase Breaker1 : spsThreePhaseBreakerLib/Three-Phase Breaker  InitialState=closed  SwitchA=on  SwitchB=on  SwitchC=on  SwitchTimes=[17]  External=on  BreakerResistance=0.01  SnubberResistance=1e6  SnubberCapacitance=inf  Measurements=None
  Three-Phase Breaker2 : spsThreePhaseBreakerLib/Three-Phase Breaker  InitialState=closed  SwitchA=on  SwitchB=on  SwitchC=on  SwitchTimes=[17]  External=on  BreakerResistance=0.01  SnubberResistance=1e6  SnubberCapacitance=inf  Measurements=None
  Three-Phase Breaker3 : spsThreePhaseBreakerLib/Three-Phase Breaker  InitialState=open  SwitchA=on  SwitchB=on  SwitchC=on  SwitchTimes=[100]  External=on  BreakerResistance=0.01  SnubberResistance=1e6  SnubberCapacitance=inf  Measurements=None
  To Workspace : ToWorkspace  VariableName=simout  SaveFormat=Timeseries  SampleTime=-1
  Turbine & Regulators M1 : Subsystem
  Turbine & Regulators M2 : Subsystem
  Turbine & Regulators M3 : Subsystem
  Variable Time Delay : VariableTransportDelay  MaximumDelay=100
  Vref1 1 : Constant  Value=1.6922
  Vref2 : Constant
  powergui : spspowerguiLib/powergui  Priority=1  SimulationMode=Discrete  SampleTime=5e-6  frequency=60  Iterations=50  frequencyindice=60  Pbase=120e6  ErrMax=0.0001  UnitsV=kV  UnitsW=MW  buscounter=0  FunctionMessages=off  echomessages=off  EnableUseOfTLC=off  CurrentSourceSwitches=off  DisableSnubberDevices=off  DisableRonSwitches=off  DisableVfSwitches=off  DisplayEquations=off  AutomaticDiscreteSolvers=off  SolverType=Tustin/Backward Euler (TBE)  Interpol=off  ExternalGateDelay=off  methode=off  Ts=100  x0status=blocks  SPID=on  SwTol=0  HookPort=off  NonlinearTolerance=1e-4  nMaxIteration=100  ContinueOnMaxIteration=off  RestoreLinks=warning  ResistiveCurrentMeasurement=off  Frange=[0:2:500]  Ylog=off  Xlog=on  ShowGrid=off  save=off  variable=ZData  structure=0  ZoomFFT=off  StartTime=0.0  cycles=1  DisplayStyle=1  fundamental=60  FreqAxis=off  MaxFrequency=1000  frequencyindicesteady=1  RmsSteady=1  display=off
  frequency_upperlimit : Outport
  frequency_lowerlimit : Outport  Port=2
  voltage_norm : Outport  Port=3
  area : Outport  Port=4
  dv/dt : Outport  Port=5
  cost : Outport  Port=6
  wires:
  "PMU (PLL-Based, Positive-Sequence)11"/3 -> [f12]
  "PMU (PLL-Based, Positive-Sequence)4"/3 -> [f4]
  MATLAB Function3/1(y) -> frequency_upperlimit/1
  Constant11/1 -> Switch1/3
  Gain/1 -> Sum5/2
  Constant12/1 -> Product/2
  MATLAB Function4/1(y) -> Gain1/1
  Bus Creator1/1 -> Reshape2/1
  "PMU (PLL-Based, Positive-Sequence)"/3 -> [f8]
  DoS/1 -> Switch1/2
  "PMU (PLL-Based, Positive-Sequence)7"/3 -> [f6]
  "PMU (PLL-Based, Positive-Sequence)13"/3 -> [f14]
  "PMU (PLL-Based, Positive-Sequence)8"/3 -> [f9]
  Product/1 -> MATLAB Function4/1(u)
  Sum/1 -> Turbine & Regulators M3/2(Pref)
  Turbine & Regulators M2/2(Vf) -> Sum8/1
  "PMU (PLL-Based, Positive-Sequence)10"/3 -> [f11]
  Bus Selector1/2 -> Scope4/1  "<Electrical power  Pe (pu)>"
  Fcn3/1 -> Scope2/1
  Turbine & Regulators M2/1(Pm) -> Synchronous Machine pu Standard/1
  Bus Selector2/1 -> Fcn3/1  "<Rotor speed deviation  dw (pu)>"
  "PMU (PLL-Based, Positive-Sequence)11"/1 -> [v12]
  "PMU (PLL-Based, Positive-Sequence)12"/2 -> [t13]
  "PMU (PLL-Based, Positive-Sequence)6"/3 -> [f5]
  Gain1/1 -> frequency_lowerlimit/1
  "PMU (PLL-Based, Positive-Sequence)10"/2 -> [t11]
  "PMU (PLL-Based, Positive-Sequence)9"/2 -> [t10]
  PID Controller1/1 -> Sum1/2, Sum2/2
  Sum8/1 -> Synchronous Machine pu Standard/2
  "PMU (PLL-Based, Positive-Sequence)1"/1 -> [v2]
  "PMU (PLL-Based, Positive-Sequence)9"/1 -> [v10]
  Three-Phase V-I Measurement1/1 -> "PMU (PLL-Based, Positive-Sequence)1"/1
  "PMU (PLL-Based, Positive-Sequence)6"/2 -> [t5]
  Fcn1/1 -> Scope3/1  "<Rotor speed deviation  dw (pu)>"
  "PMU (PLL-Based, Positive-Sequence)"/1 -> [v8]
  "PMU (PLL-Based, Positive-Sequence)4"/2 -> [t4]
  "PMU (PLL-Based, Positive-Sequence)4"/1 -> [v4]
  "PMU (PLL-Based, Positive-Sequence)1"/2 -> [t2]
  Turbine & Regulators M3/2(Vf) -> Synchronous Machine pu Standard2/2
  Three-Phase V-I Measurement4/1 -> "PMU (PLL-Based, Positive-Sequence)4"/1
  "PMU (PLL-Based, Positive-Sequence)3"/2 -> [t3]
  "PMU (PLL-Based, Positive-Sequence)7"/2 -> [t6]
  Sum3/1 -> Thermostat/1(Terr)  "Terr"
  Three-Phase V-I Measurement15/1 -> Scope9/1
  Sum2/1 -> Turbine & Regulators M2/2(Pref)
  "PMU (PLL-Based, Positive-Sequence)3"/3 -> [f3]
  Celsius to Fahrenheit/1 -> Bus Creator2/1  "Tindoors"
  Bus to Vector/1 -> 3-Phase Dynamic Load/1
  "PMU (PLL-Based, Positive-Sequence)2"/2 -> [t1]
  "PMU (PLL-Based, Positive-Sequence)8"/2 -> [t9]
  Bus Creator4/1 -> Product/1, MATLAB Function3/1(u)
  Heater/1(HeatFlow) -> Scope13/1, Integrator/1, House/1(Heater QDot In)
  Set Point/1 -> "Fahrenheit to Celsius "/1
  Three-Phase V-I Measurement9/1 -> "PMU (PLL-Based, Positive-Sequence)9"/1
  Bus Creator2/1 -> PlotResults/2  "Temperatures"
  Three-Phase V-I Measurement2/1 -> "PMU (PLL-Based, Positive-Sequence)2"/1
  Synchronous Machine pu Standard2/1 -> Bus Selector3/1, Turbine & Regulators M3/1(m)
  Bus Creator/1 -> Bus to Vector/1
  Sum4/1 -> Scope15/1, Fahrenheit to Celsius/1, Bus Creator2/2  "Toutdoors"
  Fahrenheit to Celsius/1 -> House/2(Outdoor Temp Tout)  "Tout"
  Bus Selector3/3 -> Scope7/1  "<Output active power   Peo (pu)>"
  3-Phase Dynamic Load/1 -> Bus Selector/1
  Turbine & Regulators M3/1(Pm) -> Synchronous Machine pu Standard2/1
  Bus Selector3/1 -> Fcn2/1, PID Controller2/1  "<Rotor speed deviation  dw (pu)>"
  Bus Selector3/2 -> Scope7/2  "<Electrical power  Pe (pu)>"
  Subtract/1 -> MATLAB Function/1(u)
  MATLAB Function1/1(y) -> voltage_norm/1, Display/1
  [t11] -> Bus Creator1/25
  Three-Phase V-I Measurement10/1 -> "PMU (PLL-Based, Positive-Sequence)10"/1
  [v4] -> Scope23/1, Bus Creator1/4
  [t8] -> Bus Creator1/22
  "PMU (PLL-Based, Positive-Sequence)8"/1 -> [v9]
  Constant7/1 -> Matrix Multiply/1
  [v1] -> Scope20/1, Bus Creator1/1
  "PMU (PLL-Based, Positive-Sequence)7"/1 -> [v6]
  [v6] -> Scope25/1, Bus Creator1/6
  "PMU (PLL-Based, Positive-Sequence)1"/3 -> [f2]
  Integrator/1 -> Cost Calculator/1
  [v5] -> Scope24/1, Bus Creator1/5
  Sum1/1 -> Turbine & Regulators M1/2(Pref)
  Constant6/1 -> Kalman Filter/4
  "PMU (PLL-Based, Positive-Sequence)11"/2 -> [t12]
  [v3] -> Scope22/1, Bus Creator1/3
  Vref1 1/1 -> Sum2/1
  Turbine & Regulators M1/1(Pm) -> Synchronous Machine pu Standard1/1
  [t10] -> Bus Creator1/24
  [t9] -> Bus Creator1/23
  [t6] -> Bus Creator1/20
  [t13] -> Bus Creator1/27
  Three-Phase V-I Measurement8/1 -> "PMU (PLL-Based, Positive-Sequence)8"/1
  [v9] -> Scope28/1, Bus Creator1/9
  [t1] -> Bus Creator1/15
  Fcn2/1 -> [F3], Scope6/1
  "PMU (PLL-Based, Positive-Sequence)5"/2 -> [t7]
  Bus Selector1/1 -> PID Controller1/1, Fcn1/1  "<Rotor speed deviation  dw (pu)>"
  Three-Phase V-I Measurement7/1 -> "PMU (PLL-Based, Positive-Sequence)7"/1
  PID Controller2/1 -> Sum/2
  [t5] -> Bus Creator1/19
  [v8] -> Scope27/1, Bus Creator1/8
  "PMU (PLL-Based, Positive-Sequence)12"/1 -> [v13]
  Kalman Filter/1 -> Matrix Multiply/2
  Thermostat/1(Blower switch) -> Heater/1(On/Off)  "blower cmd"
  Three-Phase V-I Measurement12/1 -> "PMU (PLL-Based, Positive-Sequence)12"/1
  "PMU (PLL-Based, Positive-Sequence)5"/1 -> [v7]
  "PMU (PLL-Based, Positive-Sequence)2"/3 -> [f1]
  [t2] -> Bus Creator1/16
  Synchronous Machine pu Standard/1 -> Bus Selector2/1, Turbine & Regulators M2/1(m)
  Switch1/1 -> Subtract/1, Kalman Filter/1
  Constant1/1 -> Sum1/1
  Constant4/1 -> Kalman Filter/2
  Matrix Multiply/1 -> Subtract/2
  "PMU (PLL-Based, Positive-Sequence)"/2 -> [t8]
  Synchronous Machine pu Standard1/1 -> Bus Selector1/1, Turbine & Regulators M1/1(m)
  [v11] -> Scope30/1, Bus Creator1/11
  [t12] -> Bus Creator1/26
  House/1(Room Temp Troom) -> Scope8/1, Celsius to Fahrenheit/1, Heater/2(Troom), Sum3/2
  [v10] -> Scope29/1, Bus Creator1/10
  [v2] -> Scope21/1, Bus Creator1/2
  Vref2/1 -> Turbine & Regulators M2/3(Vref)
  [v14] -> Scope33/1, Bus Creator1/14
  "PMU (PLL-Based, Positive-Sequence)9"/3 -> [f10]
  Three-Phase V-I Measurement6/1 -> "PMU (PLL-Based, Positive-Sequence)6"/1
  "PMU (PLL-Based, Positive-Sequence)6"/1 -> [v5]
  [t14] -> Bus Creator1/28
  [t7] -> Bus Creator1/21
  Constant2/1 -> Sum/1
  Three-Phase V-I Measurement5/1 -> "PMU (PLL-Based, Positive-Sequence)5"/1
  Constant3/1 -> Bus Creator/2
  Constant5/1 -> Kalman Filter/3
  [t4] -> Bus Creator1/18
  Three-Phase V-I Measurement13/1 -> "PMU (PLL-Based, Positive-Sequence)13"/1
  Three-Phase V-I Measurement11/1 -> "PMU (PLL-Based, Positive-Sequence)11"/1
  Bus Selector/1 -> Scope10/1  "<Positive-sequence voltage V (pu)>"
  "PMU (PLL-Based, Positive-Sequence)13"/2 -> [t14]
  [f13] -> Bus Creator4/13
  [f6] -> Bus Creator4/6
  MATLAB Function/1(y) -> Scope1/1
  [f10] -> Bus Creator4/10
  [f9] -> Bus Creator4/9
  Three-Phase V-I Measurement3/1 -> "PMU (PLL-Based, Positive-Sequence)3"/1
  "Fahrenheit to Celsius "/1 -> Sum3/1
  [f11] -> Bus Creator4/11
  "PMU (PLL-Based, Positive-Sequence)10"/1 -> [v11]
  [f7] -> Bus Creator4/7
  [f12] -> Bus Creator4/12
  Turbine & Regulators M1/2(Vf) -> Synchronous Machine pu Standard1/2
  [v12] -> Scope31/1, Bus Creator1/12
  [f14] -> Bus Creator4/14
  Three-Phase V-I Measurement/1 -> "PMU (PLL-Based, Positive-Sequence)"/1
  [t3] -> Bus Creator1/17
  [f4] -> Bus Creator4/4
  [v13] -> Scope32/1, Bus Creator1/13
  [f1] -> Scope19/1, Bus Creator4/1
  [f8] -> Bus Creator4/8
  "PMU (PLL-Based, Positive-Sequence)12"/3 -> [f13]
  [f2] -> Bus Creator4/2
  "PMU (PLL-Based, Positive-Sequence)5"/3 -> [f7]
  [f5] -> Bus Creator4/5
  Bus Selector2/2 -> Scope5/1  "<Electrical power  Pe (pu)>"
  "PMU (PLL-Based, Positive-Sequence)2"/1 -> [v1]
  Cost Calculator/1 -> PlotResults/1, Gain/1  "HeatCost"
  Reshape/1 -> Rate Transition1/1
  Reshape1/1 -> Rate Transition2/1
  Reshape2/1 -> MATLAB Function1/1(u), Switch1/1
  Rate Transition1/1 -> Scope12/1, Sum8/2
  Derivative/1 -> Display4/1, Scope17/1
  "PMU (PLL-Based, Positive-Sequence)13"/1 -> Derivative/1, Scope16/1, [v14]
  fdia/1 -> Reshape/1
  [f3] -> Bus Creator4/3
  [v7] -> Scope26/1, Bus Creator1/7
  [trigger] -> Three-Phase Breaker3/1, Three-Phase Breaker/1
  [trigger] -> Three-Phase Breaker2/1
  [trigger] -> Three-Phase Breaker1/1
  Bus Selector2/3 -> Scope37/1  "<Stator current  id (pu)>"
  Stair Generator/1 -> Sample and Hold/Trigger
  Sum9/1 -> MATLAB Function6/1(V_th_min)
  Constant14/1 -> Sum9/2
  Sample and Hold/1 -> dv/dt/1
  Variable Time Delay/1 -> [trigger]
  Abs/1 -> Sample and Hold/1
  Stair Generator1/1 -> Variable Time Delay/1
  "PMU (PLL-Based, Positive-Sequence)3"/1 -> Scope11/1, Sample and Hold1/1, Derivative1/1, [v3]
  Stair Generator2/1 -> Sample and Hold1/Trigger
  Sample and Hold1/1 -> MATLAB Function6/2(voltage)
  Avg Outdoor Temp/1 -> Sum4/1  "Toutdoors"
  temperature_sensor_hvac/1 -> Reshape1/1
  Daily Temp Variation/1 -> Sum4/2
  Rate Transition2/1 -> Sum4/3
  Integrator2/1 -> cost/1, area/1, To Workspace/1
  Sum5/1 -> Integrator2/1, Bus Creator/1
  Derivative1/1 -> Abs/1
  Constant/1 -> Sum5/1
  MATLAB Function6/1(time_delay) -> Variable Time Delay/2
  bias/1 -> Sum9/1
  connections:
  Bus_5/LConn6 -- Line 5_6/RConn3 -- Three-Phase V-I Measurement6/LConn3
  Bus_3/LConn3 -- Line 3_4/RConn3 -- Three-Phase V-I Measurement3/LConn3
  Synchronous Machine pu Standard/RConn3 -- Three-Phase Parallel RLC Load3/LConn3 -- 146.28/230kV/LConn3
  Bus_14/RConn6 -- Line 9_14/LConn3 -- Three-Phase V-I Measurement13/LConn3
  Three-Phase Parallel RLC Load3/LConn2 -- Synchronous Machine pu Standard/RConn2 -- 146.28/230kV/LConn2
  Bus_5/LConn4 -- Line 5_6/RConn1 -- Three-Phase V-I Measurement6/LConn1
  Line 5_6/LConn2 -- Bus_6/LConn5 -- Three-Phase V-I Measurement7/LConn2
  Line 6_12/LConn3 -- Bus_12/RConn3 -- Three-Phase V-I Measurement11/LConn3
  Line 5_6/LConn3 -- Bus_6/LConn6 -- Three-Phase V-I Measurement7/LConn3
  Three-Phase Parallel RLC Load1/LConn3 -- Synchronous Machine pu Standard1/RConn3 -- 144.21/230kV/LConn3
  Bus_5/LConn5 -- Line 5_6/RConn2 -- Three-Phase V-I Measurement6/LConn2
  Three-Phase V-I Measurement/LConn2 -- 150.42/230kV/RConn2 -- Bus_8/RConn2
  139.38/230kV/LConn1 -- Synchronous Machine pu Standard2/RConn1 -- Three-Phase Parallel RLC Load2/LConn1
  Bus_13/RConn9 -- Line 13-14/LConn1 -- Three-Phase V-I Measurement12/LConn3
  Line 6_12/LConn2 -- Bus_12/RConn2 -- Three-Phase V-I Measurement11/LConn2
  Bus_10/RConn3 -- Line 10-11/RConn3 -- Three-Phase V-I Measurement9/LConn3
  Three-Phase Breaker/LConn1 -- Three-Phase V-I Measurement15/LConn1
  Line 4_7/LConn2 -- Bus_7/LConn2 -- Three-Phase V-I Measurement5/LConn2
  Three-Phase Breaker/LConn3 -- Three-Phase V-I Measurement15/LConn3
  Three-Phase Parallel RLC Load3/LConn1 -- Synchronous Machine pu Standard/RConn1 -- 146.28/230kV/LConn1
  150.42/230kV/RConn1 -- Bus_8/RConn1 -- Three-Phase V-I Measurement/LConn1
  Three-Phase V-I Measurement3/LConn2 -- Line 3_4/RConn2 -- Bus_3/LConn2
  Three-Phase V-I Measurement8/LConn3 -- Three-Phase Breaker1/LConn3 -- Bus_9/RConn10
  Three-Phase V-I Measurement11/LConn1 -- Bus_12/RConn1 -- Line 6_12/LConn1
  Three-Phase Parallel RLC Load1/LConn1 -- Synchronous Machine pu Standard1/RConn1 -- 144.21/230kV/LConn1
  Bus_14/RConn5 -- Line 9_14/LConn2 -- Three-Phase V-I Measurement13/LConn2
  Bus_3/LConn1 -- Line 3_4/RConn1 -- Three-Phase V-I Measurement3/LConn1
  Bus_11/RConn6 -- Line 10-11/LConn1 -- Three-Phase V-I Measurement10/LConn3
  Three-Phase V-I Measurement8/LConn2 -- Bus_9/RConn11 -- Three-Phase Breaker1/LConn2
  Bus_10/RConn2 -- Line 10-11/RConn2 -- Three-Phase V-I Measurement9/LConn2
  Bus_7/LConn1 -- Line 4_7/LConn1 -- Three-Phase V-I Measurement5/LConn1
  Three-Phase Breaker/LConn2 -- Three-Phase V-I Measurement15/LConn2
  Bus_13/RConn7 -- Line 13-14/LConn3 -- Three-Phase V-I Measurement12/LConn1
  Three-Phase Parallel RLC Load2/LConn2 -- Synchronous Machine pu Standard2/RConn2 -- 139.38/230kV/LConn2
  Bus_2/LConn3 -- Line 1_2/RConn3 -- Three-Phase V-I Measurement1/LConn3
  Bus_2/LConn1 -- Line 1_2/RConn1 -- Three-Phase V-I Measurement1/LConn1
  Bus_11/RConn4 -- Line 10-11/LConn3 -- Three-Phase V-I Measurement10/LConn1
  Three-Phase V-I Measurement4/LConn2 -- Three-Phase Series RLC Load2/LConn2 -- Bus_4/RConn11
  Three-Phase Parallel RLC Load1/LConn2 -- Synchronous Machine pu Standard1/RConn2 -- 144.21/230kV/LConn2
  Bus_1/RConn1 -- Line 1_2/LConn1 -- Three-Phase V-I Measurement2/LConn1
  Bus_14/RConn4 -- Line 9_14/LConn1 -- Three-Phase V-I Measurement13/LConn1
  Bus_10/RConn1 -- Line 10-11/RConn1 -- Three-Phase V-I Measurement9/LConn1
  Bus_7/LConn3 -- Line 4_7/LConn3 -- Three-Phase V-I Measurement5/LConn3
  Bus_8/RConn3 -- 150.42/230kV/RConn3 -- Three-Phase V-I Measurement/LConn3
  Three-Phase V-I Measurement7/LConn1 -- Bus_6/LConn4 -- Line 5_6/LConn1
  Bus_13/RConn8 -- Line 13-14/LConn2 -- Three-Phase V-I Measurement12/LConn2
  Three-Phase V-I Measurement8/LConn1 -- Bus_9/RConn12 -- Three-Phase Breaker1/LConn1
  Bus_1/RConn3 -- Line 1_2/LConn3 -- Three-Phase V-I Measurement2/LConn3
  Bus_2/LConn2 -- Line 1_2/RConn2 -- Three-Phase V-I Measurement1/LConn2
  Three-Phase V-I Measurement4/LConn3 -- Three-Phase Series RLC Load2/LConn3 -- Bus_4/RConn12
  Bus_1/RConn2 -- Line 1_2/LConn2 -- Three-Phase V-I Measurement2/LConn2
  139.38/230kV/LConn3 -- Synchronous Machine pu Standard2/RConn3 -- Three-Phase Parallel RLC Load2/LConn3
  Line 3_4/LConn3 -- Bus_4/RConn9
  Three-Phase V-I Measurement10/LConn2 -- Line 10-11/LConn2 -- Bus_11/RConn5
  " "/LConn3 -- Bus_9/LConn6
  Three-Phase Series RLC Load7/LConn3 -- Bus_12/LConn3
  Three-Phase Series RLC Load3/LConn3 -- Bus_5/LConn1
  Line 6-11/RConn3 -- Bus_11/RConn3
  Line 7-8/LConn1 -- Bus_7/RConn4
  Bus_2/LConn5 -- Line 2-5/LConn2
  Line 4-5/RConn1 -- Bus_4/RConn1
  Bus_2/RConn8 -- Line 2-3/LConn2
  Line 7_9/RConn1 -- Bus_7/RConn1
  Line 7_9/LConn2 -- Bus_9/RConn8
  Bus_8/LConn2 -- Line 7-8/RConn2
  Line 2-4/RConn2 -- Bus_4/RConn5
  Line 6-11/RConn2 -- Bus_11/RConn2
  Line 4_9/RConn1 -- Bus_4/LConn1
  Synchronous condensor_3/RConn1 -- 150.42/230kV/LConn1
  Line 12-13/RConn3 -- Bus_13/RConn3
  Line 7-8/LConn2 -- Bus_7/RConn5
  Line 6_13/RConn1 -- Bus_6/RConn4
  Line 2-5/LConn3 -- Bus_2/LConn4
  Line 4_9/LConn2 -- Bus_9/RConn5
  Three-Phase Series RLC Load8/LConn2 -- Bus_13/LConn2
  Bus_13/RConn4 -- Line 6_13/LConn1
  Line 2-3/RConn2 -- Bus_3/RConn2
  146.28/230kV/RConn1 -- Bus_1/LConn3
  Line 7-8/LConn3 -- Bus_7/RConn6
  Three-Phase Series RLC Load4/LConn3 -- Bus_6/RConn12
  Line 12-13/LConn2 -- Bus_12/RConn5
  147.66/230kV/RConn2 -- Bus_6/LConn2
  147.66/230kV/RConn1 -- Bus_6/LConn1
  Line 12-13/RConn2 -- Bus_13/RConn2
  Line 1-5/LConn3 -- Bus_1/RConn4
  Line 1-5/LConn2 -- Bus_1/RConn5
  Synchronous condensor_3/RConn2 -- 150.42/230kV/LConn2
  Line 9-10/LConn3 -- Bus_10/RConn4
  146.28/230kV/RConn3 -- Bus_1/LConn1
  Line 4_9/LConn1 -- Bus_9/RConn4
  Line 6-11/LConn3 -- Bus_6/RConn9
  Line 4-5/LConn2 -- Bus_5/RConn8
  Line 6-11/RConn1 -- Bus_11/RConn1
  Bus_2/RConn9 -- Line 2-3/LConn1
  Line 2-3/RConn1 -- Bus_3/RConn1
  Line 2-4/LConn1 -- Bus_2/LConn7
  Line 6_12/RConn1 -- Bus_6/RConn1
  Line 2-4/LConn3 -- Bus_2/LConn9
  Line 1-5/LConn1 -- Bus_1/RConn6
  Line 1-5/RConn1 -- Bus_5/RConn1
  Line 2-5/LConn1 -- Bus_2/LConn6
  Line 9-10/LConn1 -- Bus_10/RConn6
  Line 2-3/RConn3 -- Bus_3/RConn3
  Line 4_7/RConn2 -- Bus_4/LConn5
  Bus_9/LConn3 -- Line 9_14/RConn3
  Three-Phase Series RLC Load4/LConn1 -- Bus_6/RConn10
  Line 6_12/RConn2 -- Bus_6/RConn2
  Three-Phase Series RLC Load/LConn3 -- Bus_2/RConn3
  Three-Phase Series RLC Load8/LConn1 -- Bus_13/LConn1
  Three-Phase Series RLC Load/LConn1 -- Bus_2/RConn1
  Line 2-5/RConn1 -- Bus_5/RConn6
  Three-Phase Series RLC Load6/LConn2 -- Bus_11/LConn2
  Bus_2/RConn7 -- Line 2-3/LConn3
  Bus_8/LConn1 -- Line 7-8/RConn1
  Line 7_9/LConn1 -- Bus_9/RConn7
  Line 2-4/LConn2 -- Bus_2/LConn8
  Synchronous condensor_2/RConn2 -- 147.66/230kV/LConn2
  Bus_13/RConn6 -- Line 6_13/LConn3
  Synchronous condensor_3/RConn3 -- 150.42/230kV/LConn3
  Bus_2/RConn5 -- 144.21/230kV/RConn2
  Bus_13/RConn5 -- Line 6_13/LConn2
  Line 4_9/RConn2 -- Bus_4/LConn2
  Three-Phase Series RLC Load4/LConn2 -- Bus_6/RConn11
  Line 6_12/RConn3 -- Bus_6/RConn3
  Line 9-10/RConn3 -- Bus_9/RConn3
  Line 9_14/RConn2 -- Bus_9/LConn2
  Line 7_9/LConn3 -- Bus_9/RConn9
  Line 2-4/RConn3 -- Bus_4/RConn6
  Line 4_7/RConn3 -- Bus_4/LConn6
  Bus_9/LConn1 -- Line 9_14/RConn1
  Line 9-10/RConn2 -- Bus_9/RConn2
  Three-Phase V-I Measurement15/RConn1 -- 3-Phase Dynamic Load/LConn1
  147.66/230kV/RConn3 -- Bus_6/LConn3
  Bus_3/RConn9 -- 139.38/230kV/RConn3
  3-Phase Dynamic Load/LConn3 -- Three-Phase V-I Measurement15/RConn3
  Line 12-13/LConn1 -- Bus_12/RConn6
  3-Phase Dynamic Load/LConn2 -- Three-Phase V-I Measurement15/RConn2
  Line 2-5/RConn3 -- Bus_5/RConn4
  Bus_3/RConn8 -- 139.38/230kV/RConn2
  Three-Phase Series RLC Load7/LConn2 -- Bus_12/LConn2
  Line 2-5/RConn2 -- Bus_5/RConn5
  Line 13-14/RConn3 -- Bus_14/RConn3
  Line 13-14/RConn1 -- Bus_14/RConn1
  Line 1-5/RConn3 -- Bus_5/RConn3
  Line 6-11/LConn2 -- Bus_6/RConn8
  Bus_2/RConn4 -- 144.21/230kV/RConn1
  Three-Phase Series RLC Load5/LConn3 -- Bus_10/LConn3
  Line 9-10/RConn1 -- Bus_9/RConn1
  Bus_14/RConn2 -- Line 13-14/RConn2
  Line 2-4/RConn1 -- Bus_4/RConn4
  " "/LConn1 -- Bus_9/LConn4
  Line 4-5/RConn2 -- Bus_4/RConn2
  Bus_3/RConn7 -- 139.38/230kV/RConn1
  Line 4-5/LConn1 -- Bus_5/RConn9
  Three-Phase Series RLC Load/LConn2 -- Bus_2/RConn2
  Line 12-13/LConn3 -- Bus_12/RConn4
  Three-Phase Series RLC Load5/LConn2 -- Bus_10/LConn2
  Bus_8/LConn3 -- Line 7-8/RConn3
  Line 7_9/RConn2 -- Bus_7/RConn2
  Line 4_9/RConn3 -- Bus_4/LConn3
  Line 12-13/RConn1 -- Bus_13/RConn1
  Bus_2/RConn6 -- 144.21/230kV/RConn3
  Three-Phase Series RLC Load3/LConn1 -- Bus_5/LConn3
  Line 7_9/RConn3 -- Bus_7/RConn3
  Synchronous condensor_2/RConn3 -- 147.66/230kV/LConn3
  Line 4-5/LConn3 -- Bus_5/RConn7
  Line 6_13/RConn2 -- Bus_6/RConn5
  Three-Phase Series RLC Load8/LConn3 -- Bus_13/LConn3
  Synchronous condensor_2/RConn1 -- 147.66/230kV/LConn1
  Three-Phase Series RLC Load6/LConn1 -- Bus_11/LConn1
  Three-Phase Series RLC Load3/LConn2 -- Bus_5/LConn2
  146.28/230kV/RConn2 -- Bus_1/LConn2
  Three-Phase Series RLC Load5/LConn1 -- Bus_10/LConn1
  Three-Phase Series RLC Load6/LConn3 -- Bus_11/LConn3
  Line 1-5/RConn2 -- Bus_5/RConn2
  Line 6-11/LConn1 -- Bus_6/RConn7
  Three-Phase Series RLC Load7/LConn1 -- Bus_12/LConn1
  " "/LConn2 -- Bus_9/LConn5
  Line 4_9/LConn3 -- Bus_9/RConn6
  Line 4-5/RConn3 -- Bus_4/RConn3
  Line 9-10/LConn2 -- Bus_10/RConn5
  Line 4_7/RConn1 -- Bus_4/LConn4
  Line 6_13/RConn3 -- Bus_6/RConn6
  Three-Phase Breaker/RConn3 -- Three-Phase Breaker3/RConn3 -- Bus_3/RConn6
  Three-Phase Breaker/RConn2 -- Three-Phase Breaker3/RConn2 -- Bus_3/RConn5
  Three-Phase Breaker/RConn1 -- Three-Phase Breaker3/RConn1 -- Bus_3/RConn4
  Three-Phase Breaker1/RConn1 -- Three-Phase Series RLC Load10/LConn1
  Three-Phase Breaker1/RConn2 -- Three-Phase Series RLC Load10/LConn2
  Three-Phase Breaker1/RConn3 -- Three-Phase Series RLC Load10/LConn3
  Three-Phase Breaker2/RConn1 -- Three-Phase Series RLC Load9/LConn1
  Three-Phase Breaker2/LConn2 -- Bus_14/LConn2
  Bus_14/LConn1 -- Three-Phase Breaker2/LConn1
  Bus_14/LConn3 -- Three-Phase Breaker2/LConn3
  Three-Phase Breaker2/RConn2 -- Three-Phase Series RLC Load9/LConn2
  Three-Phase Breaker2/RConn3 -- Three-Phase Series RLC Load9/LConn3
  Bus_4/RConn7 -- Line 3_4/LConn1
  Bus_4/RConn8 -- Line 3_4/LConn2
  Three-Phase V-I Measurement4/LConn1 -- Three-Phase Series RLC Load2/LConn1 -- Bus_4/RConn10
  Synchronous condensor_1/RConn3 -- 150.42/230kV1/LConn3
  Synchronous condensor_1/RConn1 -- 150.42/230kV1/LConn1
  Synchronous condensor_1/RConn2 -- 150.42/230kV1/LConn2
  Three-Phase Breaker3/LConn2 -- Three-Phase Series RLC Load13/LConn2 -- 150.42/230kV1/RConn2
  150.42/230kV1/RConn1 -- Three-Phase Series RLC Load13/LConn1 -- Three-Phase Breaker3/LConn1
  150.42/230kV1/RConn3 -- Three-Phase Series RLC Load13/LConn3 -- Three-Phase Breaker3/LConn3
